simulink model "totalSystem"  (R2013a)
settings: Solver=ode45  StartTime=0.0  StopTime=10.0  RelTol=1e-3
libraries: simulink x1
settings Model: Creator=Labo  LastModifiedBy=Labo

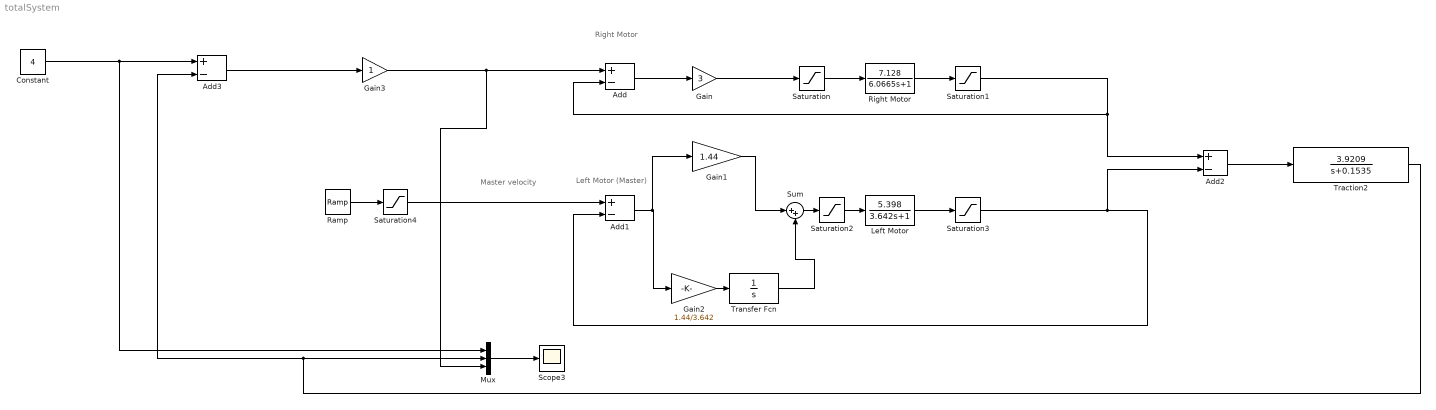
== system totalSystem ==
  note: Master velocity
  note: Left Motor (Master)
  note: Right Motor
  Add{,1..3} (4 alike) : Sum  Inputs=+-
  Constant : Constant  Value=4
  Gain : Gain  Gain=3
  Gain1 : Gain  Gain=1.44
  Gain2 : Gain  Gain=1.44/3.642
  Gain3 : Gain
  "Left Motor " : TransferFcn  Numerator=[5.398]  Denominator=[3.642 1]  ContinuousStateAttributes='v'
  Mux : Mux  Inputs=3
  Ramp : simulink/Sources/Ramp  slope=2/8  start=0  X0=0
  "Right Motor " : TransferFcn  Numerator=[7.128]  Denominator=[6.0665 1]  ContinuousStateAttributes='v'
  Saturation : Saturate  UpperLimit=7.3  LowerLimit=-17.3
  Saturation1 : Saturate  UpperLimit=10-2.79  LowerLimit=-10-2.79
  Saturation2 : Saturate  UpperLimit=7.3  LowerLimit=-17.3
  Saturation3 : Saturate  UpperLimit=10-8.623  LowerLimit=-10-8.623
  Saturation4 : Saturate  UpperLimit=2  LowerLimit=0
  Scope3 : Scope
  Sum : Sum  Inputs=|++
  Traction2 : TransferFcn  Numerator=[ 3.9209]  Denominator=[1 0.1535]
  Transfer Fcn : TransferFcn  Denominator=[1 0]
  wires:
  Add/1 -> Gain/1
  "Right Motor "/1 -> Saturation1/1
  Saturation1/1 -> Add2/1, Add/2
  Saturation/1 -> "Right Motor "/1
  Add1/1 -> Gain2/1, Gain1/1
  "Left Motor "/1 -> Saturation3/1
  Saturation3/1 -> Add1/2, Add2/2
  Saturation2/1 -> "Left Motor "/1
  Sum/1 -> Saturation2/1
  Traction2/1 -> Mux/2, Add3/2
  Constant/1 -> Add3/1, Mux/1
  Saturation4/1 -> Add1/1
  Mux/1 -> Scope3/1
  Add2/1 -> Traction2/1
  Gain2/1 -> Transfer Fcn/1
  Transfer Fcn/1 -> Sum/2
  Gain1/1 -> Sum/1
  Ramp/1 -> Saturation4/1
  Add3/1 -> Gain3/1
  Gain3/1 -> Mux/3, Add/1
  Gain/1 -> Saturation/1
